simulink model "stp1_7sym"  (R2022b)
settings: Solver=VariableStepAuto  StartTime=0.0  StopTime=20  RelTol=1e-3
values from neighbouring files (symbols this model uses):
  K = inv(M'*M + lambda*eye(Nu)) * M'    [dmc.m]    (also in dpid.m = 7.7; gpc.m; stp1.m = acker(A, B, [s s s]))
  L = acker(A', C', [s0 s0 s0])    [stp1.m]
  x1_05 = 2    [stp1.m]
  x2_05 = 1    [stp1.m]
  x3_05 = -1    [stp1.m]
  x_ob = [0 0 0]    [stp1.m]
settings Model: Creator=zalew  LastModifiedBy=zalew

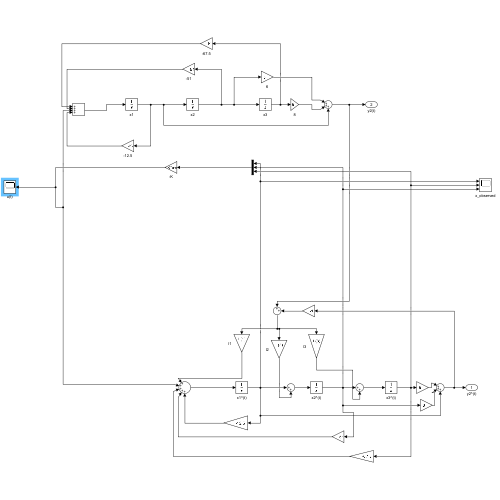
[thumbnail: Simulink's stored preview of the top-level diagram]
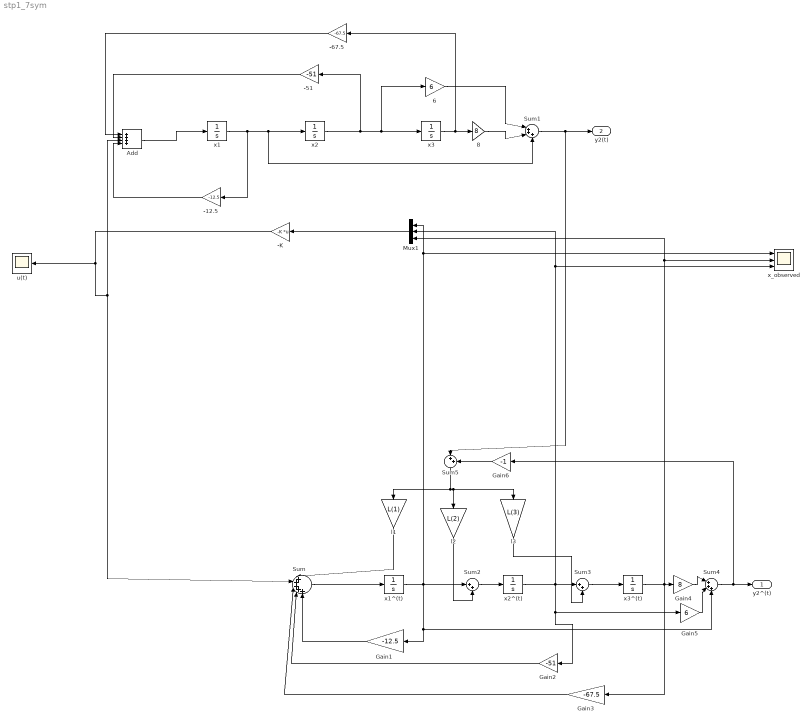
== system stp1_7sym ==
  -12.5 : Gain  Gain=-12.5
  -51 : Gain  Gain=-51
  -67.5 : Gain  Gain=-67.5
  -K : Gain  Gain=-K  Multiplication=Matrix(K*u) (u vector)
  6 : Gain  Gain=6
  8 : Gain  Gain=8
  Add : Sum  Inputs=++++
  Gain1 : Gain  Gain=-12.5
  Gain2 : Gain  Gain=-51
  Gain3 : Gain  Gain=-67.5
  Gain4 : Gain  Gain=8
  Gain5 : Gain  Gain=6
  Gain6 : Gain  Gain=-1
  Mux1 : Mux  Inputs=3
  Sum : Sum  Inputs=|+++++
  Sum1 : Sum  Inputs=|+++
  Sum2 : Sum  Inputs=|++
  Sum3 : Sum  Inputs=|++
  Sum4 : Sum  Inputs=|+++
  Sum5 : Sum  Inputs=|++
  l1 : Gain  Gain=L(1)
  l2 : Gain  Gain=L(2)
  l3 : Gain  Gain=L(3)
  u(t) : Scope
  x1 : Integrator  InitialCondition=x1_05
  x1^(t) : Integrator  InitialCondition=x_ob(1)
  x2 : Integrator  InitialCondition=x2_05
  x2^(t) : Integrator  InitialCondition=x_ob(2)
  x3 : Integrator  InitialCondition=x3_05
  x3^(t) : Integrator  InitialCondition=x_ob(3)
  x_observed : Scope  NumInputPorts=3
  y2^(t) : Outport
  y2(t) : Outport  Port=2
  wires:
  Mux1/1 -> -K/1
  Sum3/1 -> x3^(t)/1
  Sum5/1 -> l3/1, l2/1, l1/1
  Sum4/1 -> Gain6/1, y2^(t)/1
  l2/1 -> Sum2/2
  Gain1/1 -> Sum/5
  l1/1 -> Sum/1
  x2^(t)/1 -> Mux1/2, x_observed/3, Gain5/1, Gain2/1, Sum3/1
  Sum/1 -> x1^(t)/1
  l3/1 -> Sum3/2
  -67.5/1 -> Add/1
  -12.5/1 -> Add/4
  -51/1 -> Add/2
  6/1 -> Sum1/1
  Gain2/1 -> Sum/4
  x1^(t)/1 -> Mux1/1, x_observed/1, Sum4/3, Gain1/1, Sum2/1
  -K/1 -> Add/3, Sum/2, u(t)/1
  Sum1/1 -> y2(t)/1, Sum5/1
  Gain5/1 -> Sum4/2
  x3/1 -> -67.5/1, 8/1
  Gain4/1 -> Sum4/1
  x2/1 -> x3/1, 6/1, -51/1
  x1/1 -> -12.5/1, x2/1, Sum1/3
  Sum2/1 -> x2^(t)/1
  Add/1 -> x1/1
  8/1 -> Sum1/2
  Gain3/1 -> Sum/3
  Gain6/1 -> Sum5/2
  x3^(t)/1 -> x_observed/2, Mux1/3, Gain3/1, Gain4/1
